simulink model "Blog_share_ConstPowerLoad"  (R2023a)
settings: Solver=VariableStepAuto  StartTime=0.0  StopTime=100  RelTol=1e-3
InitFcn:
  | P_B = 100e6;
  | P = 1;
  | V1 = 25e3;
  | V2 = 220e3;
  | V3 = 10.5e3;
libraries: spsThreePhaseTransformerTwoWindingsLib x6, spsPower3phPhasorLib x4, spsThreePhaseParallelRLCLoadLib x4, spsThreePhaseVIMeasurementLib x4, spsThreePhaseSourceLib x4, spsThreePhasePISectionLineLib x2, spsThreePhaseDynamicLoadLib x1, sps_lib x1
settings Model: Creator=97033  LastModifiedBy=97033

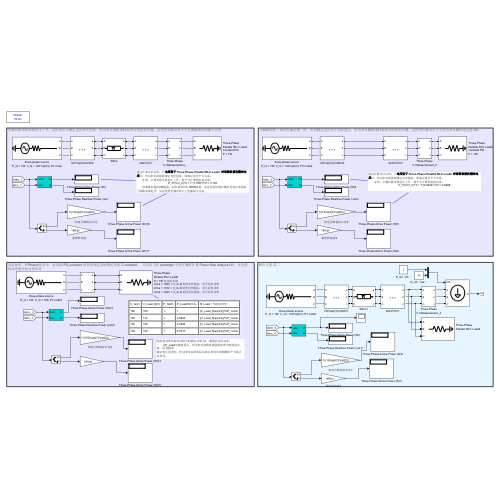
[thumbnail: Simulink's stored preview of the top-level diagram]
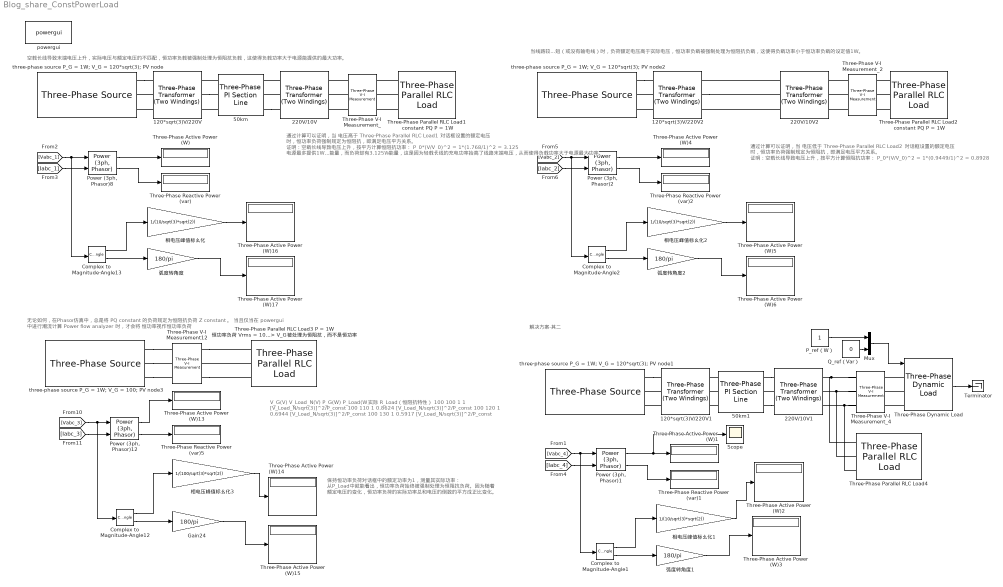
== system Blog_share_ConstPowerLoad ==
  note: 解决方案-其二
  note: 无论如何，在Phasor仿真中，总是将 PQ constant 的负荷规定为恒阻抗负荷 Z constant 。 当且仅当在 powergui 中进行潮流计算 Power flow analyzer 时，才会将
      | 恒功率视作恒功率负荷
  note: 保持恒功率负荷对话框中的额定功率为1，测量其实际功率：
      | 	从P_Load中就能看出，恒功率负荷始终被强制处理为恒阻抗负荷。因为随着
      | 额定电压的变化，恒功率负荷的实际功率总和电压的倒数的平方成正比变化。
  note: V_G(V)
      | V_Load_N(V)
      | P_G(W)
      | P_Load(W)实际
      | R_Load（恒阻抗特性）
      |
      | 100
      | 100
      | 1
      | 1
      | [V_Load_N/sqrt(3)]^2/P_const
      |
      | 100
      | 110
      | 1
      | 0.8624
      | [V_Load_N/sqrt(3)]^2/P_const
      |
      | 100
      | 120
      | 1
      | 0.6944
      | [V_Load_N/sqrt(3)]^2/P_const
      |
      | 100
      | 130
      | 1
      | 0.5917
      | [V_Load_N/sqrt(3)]^2/P_const
  note: 当线路较短（或没有输电线）时，负荷额定电压高于实际电压，恒功率负载被强制处理为恒阻抗负载，这使得负载功率小于恒功率负载的设定值1W。
  note: 空载长线导致末端电压上升，实际电压与额定电压的不匹配，恒功率负载被强制处理为恒阻抗负载，这使得负载功率大于电源能提供的最大功率。
  note: 通过计算可以证明，当 电压高于 Three-Phase Parallel RLC Load1 对话框设置的额定电压 时，恒功率负荷强制规定为恒阻抗，即满足电压平方关系。
      | 证明：空载长线导致电压上升，按平方计算恒阻抗功率：
      | P_0*(V/V_0)^2 = 1*(1.768/1)^2 = 3.125
      | 电源最多提供1W能量，而负荷却有3.125W能量，这是因为轻载长线的充电功率抬高了线路末端电压，从而使得负载功率大于电源最大功率。
  note: 通过计算可以证明，当 电压低于 Three-Phase Parallel RLC Load2 对话框设置的额定电压 时，恒功率负荷强制规定为恒阻抗，即满足电压平方关系。
      | 证明：空载长线导致电压上升，按平方计算恒阻抗功率：
      | P_0*(V/V_0)^2 = 1*(0.9449/1)^2 = 0.8928
  120*sqrt(3)V/220V : spsThreePhaseTransformerTwoWindingsLib/Three-Phase Transformer (Two Windings)  Winding1Connection=Yg  Winding2Connection=Yg  CoreType=Three single-phase transformers  SetSaturation=off  Hysteresis=off  DataFile='hysteresis'  SetInitialFlux=off  Measurements=None  UNITS=pu  NominalPower=[ P , 50 ]  Winding1=[ 120*sqrt(3) , 0.002 , 0.08 ]  Winding2=[220 , 0.002 , 0.08 ]  Rm=500  Lm=500  L0=0.5  Saturation=[ 0,0 ; 0.0024,1.2 ; 1.0,1.52 ]  InitialFluxes=[ 0.8 , -0.8 , 0.7 ]  BreakLoop=off  DiscreteSolver=Trapezoidal iterative  DataType=off  TransfoNumber=1
  120*sqrt(3)V/220V1 : spsThreePhaseTransformerTwoWindingsLib/Three-Phase Transformer (Two Windings)  Winding1Connection=Yg  Winding2Connection=Yg  CoreType=Three single-phase transformers  SetSaturation=off  Hysteresis=off  DataFile='hysteresis'  SetInitialFlux=off  Measurements=None  UNITS=pu  NominalPower=[ P , 50 ]  Winding1=[ 120*sqrt(3) , 0.002 , 0.08 ]  Winding2=[220 , 0.002 , 0.08 ]  Rm=500  Lm=500  L0=0.5  Saturation=[ 0,0 ; 0.0024,1.2 ; 1.0,1.52 ]  InitialFluxes=[ 0.8 , -0.8 , 0.7 ]  BreakLoop=off  DiscreteSolver=Trapezoidal iterative  DataType=off  TransfoNumber=1
  120*sqrt(3)V/220V2 : spsThreePhaseTransformerTwoWindingsLib/Three-Phase Transformer (Two Windings)  Winding1Connection=Yg  Winding2Connection=Yg  CoreType=Three single-phase transformers  SetSaturation=off  Hysteresis=off  DataFile='hysteresis'  SetInitialFlux=off  Measurements=None  UNITS=pu  NominalPower=[ P , 50 ]  Winding1=[ 120*sqrt(3) , 0.002 , 0.08 ]  Winding2=[220 , 0.002 , 0.08 ]  Rm=500  Lm=500  L0=0.5  Saturation=[ 0,0 ; 0.0024,1.2 ; 1.0,1.52 ]  InitialFluxes=[ 0.8 , -0.8 , 0.7 ]  BreakLoop=off  DiscreteSolver=Trapezoidal iterative  DataType=off  TransfoNumber=1
  220V/10V : spsThreePhaseTransformerTwoWindingsLib/Three-Phase Transformer (Two Windings)  Winding1Connection=Yg  Winding2Connection=Yg  CoreType=Three single-phase transformers  SetSaturation=off  Hysteresis=off  DataFile='hysteresis'  SetInitialFlux=off  Measurements=None  UNITS=pu  NominalPower=[ P , 50 ]  Winding1=[ 220 , 0.002 , 0.08 ]  Winding2=[10 , 0.002 , 0.08 ]  Rm=500  Lm=500  L0=0.5  Saturation=[ 0,0 ; 0.0024,1.2 ; 1.0,1.52 ]  InitialFluxes=[ 0.8 , -0.8 , 0.7 ]  BreakLoop=off  DiscreteSolver=Trapezoidal iterative  DataType=off  TransfoNumber=1
  220V/10V1 : spsThreePhaseTransformerTwoWindingsLib/Three-Phase Transformer (Two Windings)  Winding1Connection=Yg  Winding2Connection=Yg  CoreType=Three single-phase transformers  SetSaturation=off  Hysteresis=off  DataFile='hysteresis'  SetInitialFlux=off  Measurements=None  UNITS=pu  NominalPower=[ P , 50 ]  Winding1=[ 220 , 0.002 , 0.08 ]  Winding2=[10 , 0.002 , 0.08 ]  Rm=500  Lm=500  L0=0.5  Saturation=[ 0,0 ; 0.0024,1.2 ; 1.0,1.52 ]  InitialFluxes=[ 0.8 , -0.8 , 0.7 ]  BreakLoop=off  DiscreteSolver=Trapezoidal iterative  DataType=off  TransfoNumber=1
  220V/10V2 : spsThreePhaseTransformerTwoWindingsLib/Three-Phase Transformer (Two Windings)  Winding1Connection=Yg  Winding2Connection=Yg  CoreType=Three single-phase transformers  SetSaturation=off  Hysteresis=off  DataFile='hysteresis'  SetInitialFlux=off  Measurements=None  UNITS=pu  NominalPower=[ P , 50 ]  Winding1=[ 220 , 0.002 , 0.08 ]  Winding2=[10 , 0.002 , 0.08 ]  Rm=500  Lm=500  L0=0.5  Saturation=[ 0,0 ; 0.0024,1.2 ; 1.0,1.52 ]  InitialFluxes=[ 0.8 , -0.8 , 0.7 ]  BreakLoop=off  DiscreteSolver=Trapezoidal iterative  DataType=off  TransfoNumber=1
  50km : spsThreePhasePISectionLineLib/Three-Phase PI Section Line  LConnTagsString=a|b|c  RConnTagsString=A|B|C  Length=50  Frequency=50  Resistances=[ 0.01273 0.3864]  Inductances="[ 0.9337e-3  4.1264e-3]"  Capacitances=[12.74e-9 7.751e-9]
  50km1 : spsThreePhasePISectionLineLib/Three-Phase PI Section Line  LConnTagsString=a|b|c  RConnTagsString=A|B|C  Length=50  Frequency=50  Resistances=[ 0.01273 0.3864]  Inductances="[ 0.9337e-3  4.1264e-3]"  Capacitances=[12.74e-9 7.751e-9]
  Complex to Magnitude-Angle{1..2,12..13} (4 alike) : ComplexToMagnitudeAngle
  Gain24 : Gain  Gain=180/pi
  Mux : Mux  Inputs=2
  P_ref（W） : Constant
  Power (3ph, Phasor){1..2,8,12} (4 alike) : spsPower3phPhasorLib/Power (3ph, Phasor)
  Q_ref（Var） : Constant  Value=0
  Scope : Scope
  Terminator : Terminator
  Three-Phase Dynamic Load : spsThreePhaseDynamicLoadLib/Three-Phase Dynamic Load  NominalVoltage=[ 10 50 ]  ActiveReactivePowers=[1 0]  PositiveSequence=[0.994 -11.8]  ExternalControl=on  NpNq=[1.3 2]  TimeConstants="[0  0  0  0]"  MinimumVoltage=0.7  Tfilter=1e-4  LoadFlowParameters=[4,0,0,0,0]
      settings: LibrarySourceBlock=|
      | sps_lib/Passives/Three-Phase
      | Dynamic Load
  Three-Phase Parallel RLC Load1 constant PQ P = 1W : spsThreePhaseParallelRLCLoadLib/Three-Phase Parallel RLC Load  LConnTagsString=A|B|C  Configuration=Y (grounded)  NominalVoltage=10  Vabc=[1e3 1e3 1e3]  Vabcp=[1e3 1e3 1e3]  NominalFrequency=50  UnbalancedPower=off  ActivePower=P  InductivePower=0  CapacitivePower=0  Pabc=[10e3 9e3 11e3]  QLabc=[100 90 110]  QCabc=[100 90 110]  Pabcp=[10e3 9e3 11e3]  QLabcp=[100 90 110]  QCabcp=[100 90 110]  Measurements=None  LoadType=constant PQ
  Three-Phase Parallel RLC Load2 constant PQ P = 1W : spsThreePhaseParallelRLCLoadLib/Three-Phase Parallel RLC Load  LConnTagsString=A|B|C  Configuration=Y (grounded)  NominalVoltage=10  Vabc=[1e3 1e3 1e3]  Vabcp=[1e3 1e3 1e3]  NominalFrequency=50  UnbalancedPower=off  ActivePower=1  InductivePower=0  CapacitivePower=0  Pabc=[10e3 9e3 11e3]  QLabc=[100 90 110]  QCabc=[100 90 110]  Pabcp=[10e3 9e3 11e3]  QLabcp=[100 90 110]  QCabcp=[100 90 110]  Measurements=None  LoadType=constant PQ
  Three-Phase Parallel RLC Load3 P = 1W 恒功率负荷 Vrms = 100V = V_G 被处理为恒阻抗，而不是恒功率 Vrms = 110V > V_G 被处理为恒阻抗，而不是恒功率 Vrms = 120V > V_G 被处理为恒阻抗，而不是恒功率 : spsThreePhaseParallelRLCLoadLib/Three-Phase Parallel RLC Load  LConnTagsString=A|B|C  Configuration=Y (grounded)  NominalVoltage=130  Vabc=[1e3 1e3 1e3]  Vabcp=[1e3 1e3 1e3]  NominalFrequency=50  UnbalancedPower=off  ActivePower=P  InductivePower=0  CapacitivePower=0  Pabc=[10e3 9e3 11e3]  QLabc=[100 90 110]  QCabc=[100 90 110]  Pabcp=[10e3 9e3 11e3]  QLabcp=[100 90 110]  QCabcp=[100 90 110]  Measurements=None  LoadType=constant PQ
  "Three-Phase Parallel RLC Load4 " : spsThreePhaseParallelRLCLoadLib/Three-Phase Parallel RLC Load  LConnTagsString=A|B|C  Configuration=Y (grounded)  NominalVoltage=10  Vabc=[1e3 1e3 1e3]  Vabcp=[1e3 1e3 1e3]  NominalFrequency=50  UnbalancedPower=off  ActivePower=0.001  InductivePower=0  CapacitivePower=0  Pabc=[10e3 9e3 11e3]  QLabc=[100 90 110]  QCabc=[100 90 110]  Pabcp=[10e3 9e3 11e3]  QLabcp=[100 90 110]  QCabcp=[100 90 110]  Measurements=None  LoadType=constant Z
  Three-Phase V-I Measurement12 : spsThreePhaseVIMeasurementLib/Three-Phase V-I Measurement  VoltageMeasurement=phase-to-ground  SetLabelV=on  LabelV=Vabc_3  Vpu=off  VpuLL=off  CurrentMeasurement=yes  SetLabelI=on  LabelI=Iabc_3  Ipu=off  Pbase=100e6  Vbase=500e3  OutputType=Complex  PhasorSimulation=on  PSBequivalent=0
  Three-Phase V-I Measurement_ : spsThreePhaseVIMeasurementLib/Three-Phase V-I Measurement  VoltageMeasurement=phase-to-ground  SetLabelV=on  LabelV=Vabc_1  Vpu=off  VpuLL=off  CurrentMeasurement=yes  SetLabelI=on  LabelI=Iabc_1  Ipu=off  Pbase=100e6  Vbase=500e3  OutputType=Complex  PhasorSimulation=on  PSBequivalent=0
  Three-Phase V-I Measurement_2 : spsThreePhaseVIMeasurementLib/Three-Phase V-I Measurement  VoltageMeasurement=phase-to-ground  SetLabelV=on  LabelV=Vabc_2  Vpu=off  VpuLL=off  CurrentMeasurement=yes  SetLabelI=on  LabelI=Iabc_2  Ipu=off  Pbase=100e6  Vbase=500e3  OutputType=Complex  PhasorSimulation=on  PSBequivalent=0
  Three-Phase V-I Measurement_4 : spsThreePhaseVIMeasurementLib/Three-Phase V-I Measurement  VoltageMeasurement=phase-to-ground  SetLabelV=on  LabelV=Vabc_4  Vpu=off  VpuLL=off  CurrentMeasurement=yes  SetLabelI=on  LabelI=Iabc_4  Ipu=off  Pbase=100e6  Vbase=500e3  OutputType=Complex  PhasorSimulation=on  PSBequivalent=0
  Three-Phase Active Power (W){,1..6,13..17} (12 alike) : Display
  Three-Phase Reactive Power (var){,1..2,5} (4 alike) : Display
  powergui : sps_lib/powergui  Priority=1  SimulationMode=Phasor  SampleTime=50e-6  frequency=50  Iterations=50  frequencyindice=50  Pbase=100e6  ErrMax=1e-4  UnitsV=kV  UnitsW=MW  buscounter=0  FunctionMessages=off  echomessages=off  EnableUseOfTLC=off  CurrentSourceSwitches=off  DisableSnubberDevices=off  DisableRonSwitches=off  DisableVfSwitches=off  DisplayEquations=off  AutomaticDiscreteSolvers=off  SolverType=Tustin/Backward Euler (TBE)  Interpol=off  ExternalGateDelay=off  methode=off  Ts=100  x0status=blocks  SPID=on  SwTol=0  HookPort=off  NonlinearTolerance=1e-4  nMaxIteration=100  ContinueOnMaxIteration=off  RestoreLinks=warning  ResistiveCurrentMeasurement=off  Frange=[0:2:500]  Ylog=off  Xlog=on  ShowGrid=off  save=off  variable=ZData  structure=0  ZoomFFT=off  StartTime=0.0  cycles=1  DisplayStyle=1  fundamental=60  FreqAxis=off  MaxFrequency=1000  frequencyindicesteady=1  RmsSteady=1  display=off
  three-phase source P_G = 1W; V_G = 100; PV node3 : spsThreePhaseSourceLib/Three-Phase Source  InternalConnection=Yg  VoltagePhases=off  Voltage=100  PhaseAngle=0  Voltage_phases=[25e3 25e3 25e3]/sqrt(3)  PhaseAngles_phases=[0 -120 +120]  Frequency=50  NonIdealSource=on  SpecifyImpedance=off  Resistance=0.09  Inductance=0  ShortCircuitLevel=100e6  BaseVoltage=120*sqrt(3)  XRratio=7  BusType=PV  Pref=P  Qref=0  Prefabc=[10e3, 10e3, 10e3]  Qrefabc=[0, 0, 0]  Qmin=-inf  Qmax=inf
  three-phase source P_G = 1W; V_G = 120*sqrt(3); PV node : spsThreePhaseSourceLib/Three-Phase Source  InternalConnection=Yg  VoltagePhases=off  Voltage=120*sqrt(3)  PhaseAngle=0  Voltage_phases=[25e3 25e3 25e3]/sqrt(3)  PhaseAngles_phases=[0 -120 +120]  Frequency=50  NonIdealSource=on  SpecifyImpedance=off  Resistance=0.09  Inductance=0  ShortCircuitLevel=100e6  BaseVoltage=120*sqrt(3)  XRratio=7  BusType=PV  Pref=P  Qref=0  Prefabc=[10e3, 10e3, 10e3]  Qrefabc=[0, 0, 0]  Qmin=-inf  Qmax=inf
  three-phase source P_G = 1W; V_G = 120*sqrt(3); PV node1 : spsThreePhaseSourceLib/Three-Phase Source  InternalConnection=Yg  VoltagePhases=off  Voltage=120*sqrt(3)  PhaseAngle=0  Voltage_phases=[25e3 25e3 25e3]/sqrt(3)  PhaseAngles_phases=[0 -120 +120]  Frequency=50  NonIdealSource=on  SpecifyImpedance=off  Resistance=0.09  Inductance=0  ShortCircuitLevel=100e6  BaseVoltage=120*sqrt(3)  XRratio=7  BusType=PV  Pref=P  Qref=0  Prefabc=[10e3, 10e3, 10e3]  Qrefabc=[0, 0, 0]  Qmin=-inf  Qmax=inf
  three-phase source P_G = 1W; V_G = 120*sqrt(3); PV node2 : spsThreePhaseSourceLib/Three-Phase Source  InternalConnection=Yg  VoltagePhases=off  Voltage=120*sqrt(3)  PhaseAngle=0  Voltage_phases=[25e3 25e3 25e3]/sqrt(3)  PhaseAngles_phases=[0 -120 +120]  Frequency=50  NonIdealSource=on  SpecifyImpedance=off  Resistance=0.09  Inductance=0  ShortCircuitLevel=100e6  BaseVoltage=120*sqrt(3)  XRratio=7  BusType=PV  Pref=P  Qref=0  Prefabc=[10e3, 10e3, 10e3]  Qrefabc=[0, 0, 0]  Qmin=-inf  Qmax=inf
  弧度转角度 : Gain  Gain=180/pi
  弧度转角度1 : Gain  Gain=180/pi
  弧度转角度2 : Gain  Gain=180/pi
  相电压峰值标幺化 : Gain  Gain=1/(10/sqrt(3)*sqrt(2))
  相电压峰值标幺化1 : Gain  Gain=1/(10/sqrt(3)*sqrt(2))
  相电压峰值标幺化2 : Gain  Gain=1/(10/sqrt(3)*sqrt(2))
  相电压峰值标幺化3 : Gain  Gain=1/(100/sqrt(3)*sqrt(2))
  wires:
  弧度转角度/1 -> Three-Phase Active Power (W)17/1
  Complex to Magnitude-Angle13/2 -> 弧度转角度/1
  相电压峰值标幺化/1 -> Three-Phase Active Power (W)16/1
  [Vabc_1] -> Complex to Magnitude-Angle13/1, "Power (3ph, Phasor)8"/1
  "Power (3ph, Phasor)8"/1 -> Three-Phase Active Power (W)/1
  "Power (3ph, Phasor)8"/2 -> Three-Phase Reactive Power (var)/1
  Complex to Magnitude-Angle13/1 -> 相电压峰值标幺化/1
  [Iabc_1] -> "Power (3ph, Phasor)8"/2
  Complex to Magnitude-Angle2/1 -> 相电压峰值标幺化2/1
  [Iabc_2] -> "Power (3ph, Phasor)2"/2
  [Vabc_2] -> Complex to Magnitude-Angle2/1, "Power (3ph, Phasor)2"/1
  相电压峰值标幺化2/1 -> Three-Phase Active Power (W)5/1
  Complex to Magnitude-Angle2/2 -> 弧度转角度2/1
  弧度转角度2/1 -> Three-Phase Active Power (W)6/1
  "Power (3ph, Phasor)2"/2 -> Three-Phase Reactive Power (var)2/1
  "Power (3ph, Phasor)2"/1 -> Three-Phase Active Power (W)4/1
  [Iabc_3] -> "Power (3ph, Phasor)12"/2
  "Power (3ph, Phasor)12"/2 -> Three-Phase Reactive Power (var)5/1
  "Power (3ph, Phasor)12"/1 -> Three-Phase Active Power (W)13/1
  [Vabc_3] -> Complex to Magnitude-Angle12/1, "Power (3ph, Phasor)12"/1
  Gain24/1 -> Three-Phase Active Power (W)15/1
  相电压峰值标幺化3/1 -> Three-Phase Active Power (W)14/1
  Complex to Magnitude-Angle12/1 -> 相电压峰值标幺化3/1
  Complex to Magnitude-Angle12/2 -> Gain24/1
  P_ref（W）/1 -> Mux/1
  Q_ref（Var）/1 -> Mux/2
  Mux/1 -> Three-Phase Dynamic Load/1
  [Vabc_4] -> Complex to Magnitude-Angle1/1, "Power (3ph, Phasor)1"/1
  Complex to Magnitude-Angle1/1 -> 相电压峰值标幺化1/1
  相电压峰值标幺化1/1 -> Three-Phase Active Power (W)2/1
  Complex to Magnitude-Angle1/2 -> 弧度转角度1/1
  "Power (3ph, Phasor)1"/2 -> Three-Phase Reactive Power (var)1/1
  弧度转角度1/1 -> Three-Phase Active Power (W)3/1
  [Iabc_4] -> "Power (3ph, Phasor)1"/2
  "Power (3ph, Phasor)1"/1 -> Scope/1, Three-Phase Active Power (W)1/1
  Three-Phase Dynamic Load/1 -> Terminator/1
  connections:
  Three-Phase Parallel RLC Load1 constant PQ P = 1W/LConn3 -- Three-Phase V-I Measurement_/RConn3
  120*sqrt(3)V/220V/LConn2 -- three-phase source P_G = 1W; V_G = 120*sqrt(3); PV node/RConn2
  Three-Phase Parallel RLC Load1 constant PQ P = 1W/LConn2 -- Three-Phase V-I Measurement_/RConn2
  120*sqrt(3)V/220V/LConn3 -- three-phase source P_G = 1W; V_G = 120*sqrt(3); PV node/RConn3
  Three-Phase V-I Measurement_/LConn2 -- 220V/10V/RConn2
  50km/LConn3 -- 120*sqrt(3)V/220V/RConn3
  120*sqrt(3)V/220V/RConn2 -- 50km/LConn2
  50km/RConn3 -- 220V/10V/LConn3
  220V/10V/LConn2 -- 50km/RConn2
  Three-Phase V-I Measurement_/LConn3 -- 220V/10V/RConn3
  Three-Phase Parallel RLC Load1 constant PQ P = 1W/LConn1 -- Three-Phase V-I Measurement_/RConn1
  Three-Phase V-I Measurement_/LConn1 -- 220V/10V/RConn1
  220V/10V/LConn1 -- 50km/RConn1
  50km/LConn1 -- 120*sqrt(3)V/220V/RConn1
  three-phase source P_G = 1W; V_G = 120*sqrt(3); PV node/RConn1 -- 120*sqrt(3)V/220V/LConn1
  Three-Phase V-I Measurement_2/LConn2 -- 220V/10V2/RConn2
  three-phase source P_G = 1W; V_G = 120*sqrt(3); PV node2/RConn1 -- 120*sqrt(3)V/220V2/LConn1
  Three-Phase V-I Measurement_2/LConn1 -- 220V/10V2/RConn1
  Three-Phase Parallel RLC Load2 constant PQ P = 1W/LConn1 -- Three-Phase V-I Measurement_2/RConn1
  120*sqrt(3)V/220V2/RConn2 -- 220V/10V2/LConn2
  Three-Phase Parallel RLC Load2 constant PQ P = 1W/LConn2 -- Three-Phase V-I Measurement_2/RConn2
  220V/10V2/LConn3 -- 120*sqrt(3)V/220V2/RConn3
  Three-Phase Parallel RLC Load2 constant PQ P = 1W/LConn3 -- Three-Phase V-I Measurement_2/RConn3
  120*sqrt(3)V/220V2/LConn3 -- three-phase source P_G = 1W; V_G = 120*sqrt(3); PV node2/RConn3
  120*sqrt(3)V/220V2/LConn2 -- three-phase source P_G = 1W; V_G = 120*sqrt(3); PV node2/RConn2
  Three-Phase V-I Measurement_2/LConn3 -- 220V/10V2/RConn3
  220V/10V2/LConn1 -- 120*sqrt(3)V/220V2/RConn1
  three-phase source P_G = 1W; V_G = 100; PV node3/RConn2 -- Three-Phase V-I Measurement12/LConn2
  Three-Phase V-I Measurement12/RConn3 -- Three-Phase Parallel RLC Load3 P = 1W 恒功率负荷 Vrms = 100V = V_G 被处理为恒阻抗，而不是恒功率 Vrms = 110V > V_G 被处理为恒阻抗，而不是恒功率 Vrms = 120V > V_G 被处理为恒阻抗，而不是恒功率/LConn3
  three-phase source P_G = 1W; V_G = 100; PV node3/RConn1 -- Three-Phase V-I Measurement12/LConn1
  three-phase source P_G = 1W; V_G = 100; PV node3/RConn3 -- Three-Phase V-I Measurement12/LConn3
  Three-Phase Parallel RLC Load3 P = 1W 恒功率负荷 Vrms = 100V = V_G 被处理为恒阻抗，而不是恒功率 Vrms = 110V > V_G 被处理为恒阻抗，而不是恒功率 Vrms = 120V > V_G 被处理为恒阻抗，而不是恒功率/LConn2 -- Three-Phase V-I Measurement12/RConn2
  Three-Phase V-I Measurement12/RConn1 -- Three-Phase Parallel RLC Load3 P = 1W 恒功率负荷 Vrms = 100V = V_G 被处理为恒阻抗，而不是恒功率 Vrms = 110V > V_G 被处理为恒阻抗，而不是恒功率 Vrms = 120V > V_G 被处理为恒阻抗，而不是恒功率/LConn1
  Three-Phase Dynamic Load/LConn1 -- Three-Phase V-I Measurement_4/RConn1
  Three-Phase V-I Measurement_4/LConn2 -- 220V/10V1/RConn2 -- "Three-Phase Parallel RLC Load4 "/LConn2
  three-phase source P_G = 1W; V_G = 120*sqrt(3); PV node1/RConn1 -- 120*sqrt(3)V/220V1/LConn1
  Three-Phase V-I Measurement_4/LConn1 -- "Three-Phase Parallel RLC Load4 "/LConn1 -- 220V/10V1/RConn1
  Three-Phase Dynamic Load/LConn2 -- Three-Phase V-I Measurement_4/RConn2
  120*sqrt(3)V/220V1/LConn3 -- three-phase source P_G = 1W; V_G = 120*sqrt(3); PV node1/RConn3
  120*sqrt(3)V/220V1/LConn2 -- three-phase source P_G = 1W; V_G = 120*sqrt(3); PV node1/RConn2
  Three-Phase V-I Measurement_4/LConn3 -- 220V/10V1/RConn3 -- "Three-Phase Parallel RLC Load4 "/LConn3
  Three-Phase Dynamic Load/LConn3 -- Three-Phase V-I Measurement_4/RConn3
  50km1/LConn1 -- 120*sqrt(3)V/220V1/RConn1
  120*sqrt(3)V/220V1/RConn2 -- 50km1/LConn2
  50km1/LConn3 -- 120*sqrt(3)V/220V1/RConn3
  50km1/RConn1 -- 220V/10V1/LConn1
  220V/10V1/LConn2 -- 50km1/RConn2
  50km1/RConn3 -- 220V/10V1/LConn3
